simulink model "DF_DOB"  (R2020a)
settings: Solver=ode1  StartTime=0.0  StopTime=10  FixedStep=0.0001  RelTol=1e-3
undefined symbols (not defined in the file): A, B, C, D, SEA
libraries: simulink x5, cstblocks x4, cjt_library_models x1
settings Model: Creator=erimc  LastModifiedBy=Erim Can Ozcinar

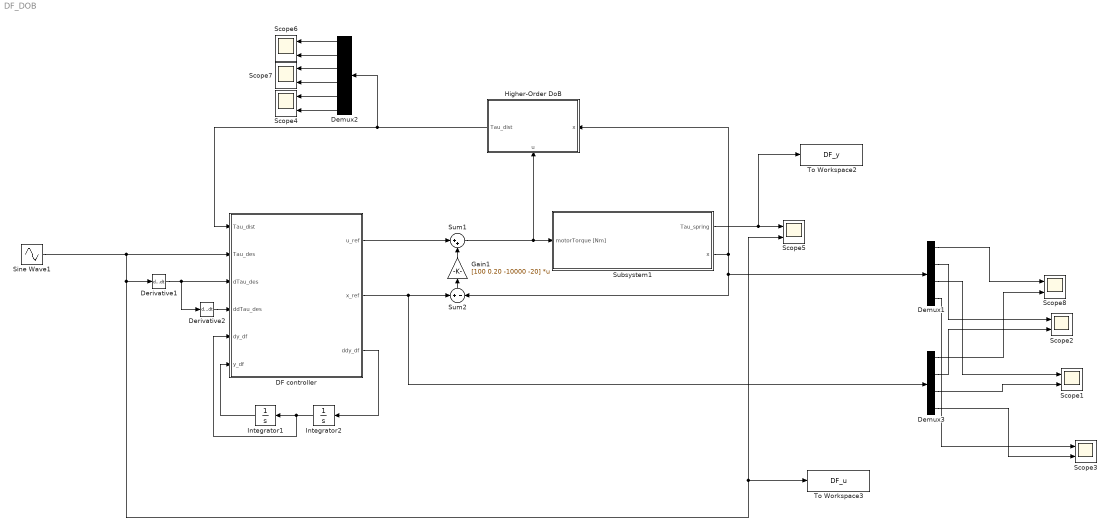
== system DF_DOB ==
  DF controller : MATLAB Function  TreatAsAtomicUnit=on
  Demux1 : Demux
  Demux2 : Demux  Outputs=6
  Demux3 : Demux
  Derivative1 : Derivative
  Derivative2 : Derivative
  Gain1 : Gain  Gain=[100 0.20 -10000 -20]  Multiplication=Matrix(K*u)
  Higher-Order DoB : Subsystem
      settings: PortSchema="{\"entries\":[{\"content\":{\"sides\":[{\"content\":{\"connectorIds\":[\"In1\"]},\"type\":\"ConnectorPlacement.EquallySpacedRectSide\",\"uuid\":\"033a9072-c968-43bf-9f71-6521bdc98383\"},{\"content\":{\"connectorIds\":[\"Out1\"],\"side\":\"RIGHT\"},\"type\":\"ConnectorPlacement.EquallySpacedRectSide\",\"uuid\":\"95ac0c33-e59d-4ac0-96cc-facae06806bd\"},{\"content\":{\"connectorIds\":[],\"side\":\"TOP\"},\"type\":\"ConnectorPlacement.EquallySpacedRectSide\",\"uuid\":\"4271cccc-922d-4503-b442-5df2d938e766\"},{\"content\":{\"connectorIds\":[\"In2\"],\"side\":\"BOTTOM\"},\"type\":\"ConnectorPlacement.EquallySpacedRectSide\",\"uuid\":\"8fe68d28-3df5-4424-a916-547538c04804\"}]},\"type\":\"ConnectorPlacement.EquallySpacedConnector\",\"uuid\":\"e60c16e9-b2aa-49f1-a4b3-0df40270c19e\"}],\"packageUris\":[\"http://schema.mathworks.com/mf0/Connector/19700101\"],\"version\":\"1.0\"}"
  Integrator1 : Integrator
  Integrator2 : Integrator
  Scope{1..8} (8 alike) : Scope  NumInputPorts=2
  Sine Wave1 : Sin  Amplitude=10  SampleTime=0
  Subsystem1 : Subsystem
  Sum1 : Sum  Inputs=|++
  Sum2 : Sum  Inputs=+|-
  To Workspace2 : ToWorkspace  VariableName=DF_y  SampleTime=-1
      settings: Save2DSignal=2-D array (concatenate along first dimension)
  To Workspace3 : ToWorkspace  VariableName=DF_u  SampleTime=-1
      settings: Save2DSignal=2-D array (concatenate along first dimension)
  wires:
  Integrator1/1 -> DF controller/6(y_df)
  Sum1/1 -> Subsystem1/1(motorTorque [Nm]), Higher-Order DoB/2(u)
  DF controller/2(x_ref) -> Sum2/1, Demux3/1
  DF controller/1(u_ref) -> Sum1/1
  Subsystem1/1(Tau_spring) -> To Workspace2/1, Scope5/1
  Demux1/1 -> Scope8/1
  Demux2/5 -> Scope4/1
  Subsystem1/2(x) -> Higher-Order DoB/1(x), Sum2/2, Demux1/1
  Demux3/3 -> Scope1/2
  Demux3/1 -> Scope8/2
  Demux3/2 -> Scope2/2
  Derivative1/1 -> DF controller/3(dTau_des), Derivative2/1
  Demux3/4 -> Scope3/2
  DF controller/3(ddy_df) -> Integrator2/1
  Demux1/2 -> Scope2/1
  Demux2/6 -> Scope4/2
  Demux2/2 -> Scope6/2
  Integrator2/1 -> DF controller/5(dy_df), Integrator1/1
  Demux1/3 -> Scope1/1
  Demux2/1 -> Scope6/1
  Demux1/4 -> Scope3/1
  Higher-Order DoB/1(Tau_dist) -> DF controller/1(Tau_dist), Demux2/1
  Demux2/3 -> Scope7/1
  Sine Wave1/1 -> DF controller/2(Tau_des), To Workspace3/1, Scope5/2, Derivative1/1
  Demux2/4 -> Scope7/2
  Gain1/1 -> Sum1/2
  Sum2/1 -> Gain1/1
  Derivative2/1 -> DF controller/4(ddTau_des)

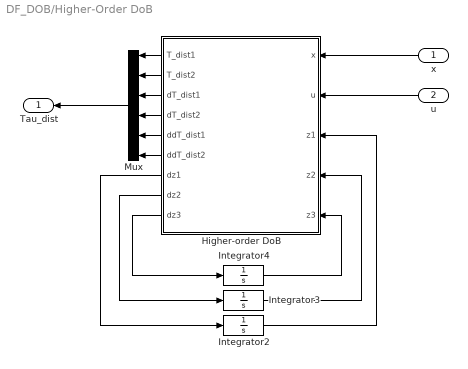
== system DF_DOB/Higher-Order DoB ==
  x : Inport
  u : Inport  Port=2
  Higher-order DoB : MATLAB Function  TreatAsAtomicUnit=on
  Integrator2 : Integrator
  Integrator3 : Integrator
  Integrator4 : Integrator
  Mux : Mux  Inputs=6
  Tau_dist : Outport
  wires:
  Integrator2/1 -> Higher-order DoB/3(z1)
  x/1 -> Higher-order DoB/1(x)
  u/1 -> Higher-order DoB/2(u)
  Integrator4/1 -> Higher-order DoB/5(z3)
  Integrator3/1 -> Higher-order DoB/4(z2)
  Higher-order DoB/1(T_dist1) -> Mux/1
  Higher-order DoB/2(T_dist2) -> Mux/2
  Higher-order DoB/3(dT_dist1) -> Mux/3
  Higher-order DoB/4(dT_dist2) -> Mux/4
  Higher-order DoB/5(ddT_dist1) -> Mux/5
  Higher-order DoB/6(ddT_dist2) -> Mux/6
  Mux/1 -> Tau_dist/1
  Higher-order DoB/8(dz2) -> Integrator3/1
  Higher-order DoB/7(dz1) -> Integrator2/1
  Higher-order DoB/9(dz3) -> Integrator4/1

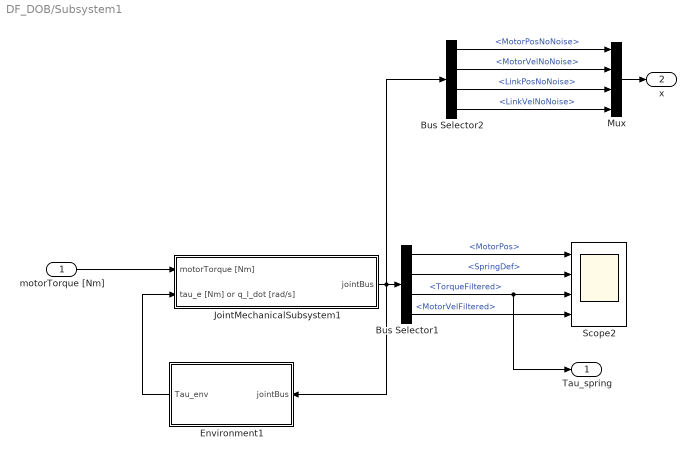
== system DF_DOB/Subsystem1 ==
  motorTorque [Nm] : Inport
  Bus Selector1 : BusSelector  OutputSignals=MotorPos,SpringDef,TorqueFiltered,MotorVelFiltered
  Bus Selector2 : BusSelector  OutputSignals=MotorPosNoNoise,MotorVelNoNoise,LinkPosNoNoise,LinkVelNoNoise
  Environment1 : Subsystem
  JointMechanicalSubsystem1 : Subsystem  AncestorBlock=cjt_library_models/Joint models/JointMechanicalSubsystem  mask(jointMechanicalSubsystem){jointObj=SEA, fc_vel=1000, fc_torque=1000, input_delay=0, output_delay=0, quantize=on, quantize_bits=19, input_noise_enabled=on, output_noise_enabled=on, var_u=0.021, var_y=1e-10}
      mask prompts: jointObj "Joint Object"; fc_vel "Velocity filter cut-off frequency [Hz]"; fc_torque "Torque filter cut-off frequency [Hz]"; input_delay "Motor torque input delay (num samples of Ts)"; output_delay "Output delay (num samples of Ts)"; quantize "Quantize measurements"; quantize_bits "Quantization bits"; input_noise_enabled "Enable input noise"; output_noise_enabled "Enable measurement noise"; var_u "Input noise variance"; var_y "Measurement noise variance"
      mask help:
      | This block implements the mechanical dynamics of the actuator.
      |
      | For more information, see the > Help <.
      mask init:
      | % Get linear dynamics matrices
      | [A, B, C, D, I, R, K] = jointObj.getDynamicsMatrices();
      | 
      | % Build B matrix for nonlinear components
      | B_nonlinear = [zeros([size(B,1)-size(I,1),1]); 1./diag(I)];
      | 
      | % Get other properties
      | Ts      = jointObj.Ts;
      | Ts_elec = jointObj.Ts_elec;
      | k_b     = jointObj.k_b;
      | k_t     = jointObj.k_t;
      | n       = jointObj.n;
      | d_gl    = jointObj.d_gl;
      | 
      | % Handle MATLAB function block
      | handleMatlabFunctionBlock(gcb, jointObj);
      | 
      | % If input delay is enabled, set the flag to 1
      | input_delay_enable = 0;
      | if (input_delay > 0)
      |     input_delay_enable = 1;
      | end
      | 
      | % If noise is disabled, overwrite the given variances
      | if (input_noise_enabled == 0)
      |     var_u = 0;
      | end
      | if (output_noise_enabled == 0)
      | 	var_y = 0;
      | end
      mask Help:
      | This block implements the mechanical dynamics of the actuator. Depending on the configuration in which the joint class was built, its dynamics are given by one of the variants provided by the toolbox (see model/linear/). If provided, the linear dynamics are enhanced with nonlinear components.
      | 
      | <b>Inputs</b>
      | <b>motorTorque</b>: Electromechanical motor torque provided on the rotor. An input delay can be added to this input (e.g. due to communication delays or a very simplified representation of electrical dynamics).
      | <b>tau_e or q_l_dot</b>: External interaction torque. Depending on the selected linear dynamics model of the joint, this is either the external torque acting on the load or the imposed load velocity (for fixed-output models).
      | 
      | <b>Outputs</b>
      | <b>jointBus</b>: The various variables and their measurements, with optional delays/noise/quantisation etc. For most outputs, several instances exist. Output variables ending in "NoNoise" denote physical quantities, without noise, filtering, or delays. All other variables are affected by noise and delays (if enabled). Lastly, variables ending in "Filtered" are also low-pass filtered, with cut-off frequency set in the mask.
      | 
      | <b>An important note with regards to output variables associated with torque.</b>
      | The "Torque" and "TorqueFiltered" are computed in the way torque is usually sensed by the control system; deflection times spring constant, i.e. only the stiffness contribution is considered, as usually the internal damping of the used flexible element (parameter d_gl) is very small. Hence, TorqueFiltered is used by the toolbox controllers as well.
      | However, as noted before, "TorqueNoNoise" denotes the physical quantity. This means that it includes the torque produced by internal damping of the elastic element (parameter d_gl).
      mask Callback quantize: toggleMaskFields(gcbh, 'quantize', 'quantize_bits');
      mask Callback input_noise_enabled: toggleMaskFields(gcbh, 'input_noise_enabled', 'var_u');
      mask Callback output_noise_enabled: toggleMaskFields(gcbh, 'output_noise_enabled', 'var_y');
  Mux : Mux
  Scope2 : Scope  NumInputPorts=4
  Tau_spring : Outport
  x : Outport  Port=2
  wires:
  Bus Selector1/2 -> Scope2/2  "<SpringDef>"
  Bus Selector1/3 -> Tau_spring/1, Scope2/3  "<TorqueFiltered>"
  JointMechanicalSubsystem1/1(jointBus) -> Bus Selector2/1, Environment1/1(jointBus), Bus Selector1/1
  Bus Selector1/1 -> Scope2/1  "<MotorPos>"
  motorTorque [Nm]/1 -> JointMechanicalSubsystem1/1(motorTorque [Nm])
  Bus Selector2/1 -> Mux/1  "<MotorPosNoNoise>"
  Bus Selector2/2 -> Mux/2  "<MotorVelNoNoise>"
  Bus Selector2/3 -> Mux/3  "<LinkPosNoNoise>"
  Bus Selector2/4 -> Mux/4  "<LinkVelNoNoise>"
  Mux/1 -> x/1
  Bus Selector1/4 -> Scope2/4  "<MotorVelFiltered>"
  Environment1/1(Tau_env) -> JointMechanicalSubsystem1/2(tau_e [Nm] or q_l_dot [rad/s])

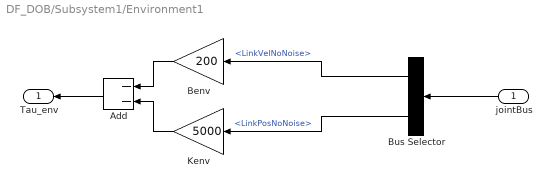
== system DF_DOB/Subsystem1/Environment1 ==
  jointBus : Inport
  Add : Sum  Inputs=--
  Benv : Gain  Gain=200
  Bus Selector : BusSelector  OutputSignals=LinkVelNoNoise,LinkPosNoNoise
  Kenv : Gain  Gain=5000
  Tau_env : Outport
  wires:
  Kenv/1 -> Add/2
  Benv/1 -> Add/1
  Add/1 -> Tau_env/1
  Bus Selector/1 -> Benv/1  "<LinkVelNoNoise>"
  Bus Selector/2 -> Kenv/1  "<LinkPosNoNoise>"
  jointBus/1 -> Bus Selector/1

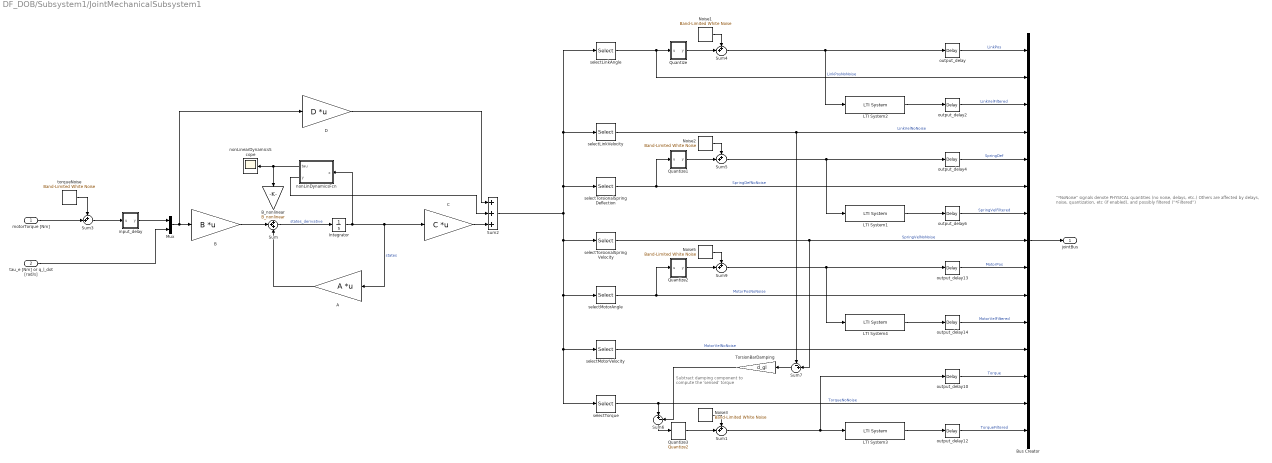
== system DF_DOB/Subsystem1/JointMechanicalSubsystem1 ==
  note: "*NoNoise" signals denote PHYSICAL quantities (no noise, delays, etc.)
      | Others are affected by delays, noise, quantization, etc (if enabled), and possibly filtered ("*Filtered")
  note: Subtract damping component to
      | compute the 'sensed' torque
  motorTorque [Nm] : Inport
  tau_e [Nm] or q_l_dot [rad/s] : Inport  Port=2
  A : Gain  Gain=A  Multiplication=Matrix(K*u)
  B : Gain  Gain=B  Multiplication=Matrix(K*u)
  B_nonlinear : Gain  Gain=B_nonlinear
  Bus Creator : BusCreator  Inputs=15
  C : Gain  Gain=C  Multiplication=Matrix(K*u)
  D : Gain  Gain=D  Multiplication=Matrix(K*u)
  Integrator : Integrator
  LTI System1 : cstblocks/LTI System  sys=c2d(tf([2*pi*fc_vel 0], [1 2*pi*fc_vel]), Ts, 'tustin')  IC=[]
  LTI System2 : cstblocks/LTI System  sys=c2d(tf([2*pi*fc_vel 0], [1 2*pi*fc_vel]), Ts, 'tustin')  IC=[]
  LTI System3 : cstblocks/LTI System  sys=c2d(tf([2*pi*fc_torque], [1 2*pi*fc_torque]), Ts, 'tustin')  IC=[]
  LTI System4 : cstblocks/LTI System  sys=c2d(tf([2*pi*fc_vel 0], [1 2*pi*fc_vel]), Ts, 'tustin')  IC=[]
  Mux : Mux  Inputs=2
  Noise1 : simulink/Sources/Band-Limited White Noise  Cov=var_y * Ts  Ts=Ts  seed=[3846513]
  Noise2 : simulink/Sources/Band-Limited White Noise  Cov=var_y * Ts  Ts=Ts  seed=[11563454]
  Noise3 : simulink/Sources/Band-Limited White Noise  Cov=sqrt(2) * var_y * Ts % sqrt(2) accounts for subtracting two encoders  Ts=Ts  seed=[960834]
  Noise5 : simulink/Sources/Band-Limited White Noise  Cov=var_y * Ts  Ts=Ts  seed=[24326]
  Quantize : Subsystem
  Quantize1 : Subsystem
  Quantize2 : Subsystem
  Quantize3 : cjt_library_models/Joint models/JointMechanicalSubsystem/Quantize2  SystemSampleTime=-1  Latency=0  AutoFrameSizeCalculation=off
  Sum : Sum  Inputs=+++
  Sum{1,3..5,9} (5 alike) : Sum  Inputs=++|
  Sum2 : Sum  Inputs=+++
  Sum6 : Sum  Inputs=|+-
  Sum7 : Sum  Inputs=-+|
  TorsionBarDamping : Gain  Gain=d_gl
  input_delay : Subsystem
  nonLinDynamicsFcn : MATLAB Function  TreatAsAtomicUnit=on
  nonLinearDynamicsScope : Scope
  output_delay{,2,4,6,10,12..14} (8 alike) : TransportDelay  DelayTime=output_delay * jointObj.Ts
  selectLinkAngle : Selector  NumberOfDimensions=2  InputPortWidth=3  IndexOptions=Index vector (dialog),Select all  Indices=3,1  OutputSizes=1,1
  selectLinkVelocity : Selector  NumberOfDimensions=2  InputPortWidth=3  IndexOptions=Index vector (dialog),Select all  Indices=6,1  OutputSizes=1,1
  selectMotorAngle : Selector  NumberOfDimensions=2  InputPortWidth=3  IndexOptions=Index vector (dialog),Select all  Indices=1,1  OutputSizes=1,1
  selectMotorVelocity : Selector  NumberOfDimensions=2  InputPortWidth=3  IndexOptions=Index vector (dialog),Select all  Indices=4,1  OutputSizes=1,1
  selectTorque : Selector  NumberOfDimensions=2  InputPortWidth=3  IndexOptions=Index vector (dialog),Select all  Indices=7,1  OutputSizes=1,1
  selectTorsionalSpringDeflection : Selector  NumberOfDimensions=2  InputPortWidth=3  IndexOptions=Index vector (dialog),Select all  Indices=2,1  OutputSizes=1,1
  selectTorsionalSpringVelocity : Selector  NumberOfDimensions=2  InputPortWidth=3  IndexOptions=Index vector (dialog),Select all  Indices=5,1  OutputSizes=1,1
  torqueNoise : simulink/Sources/Band-Limited White Noise  Cov=var_u * Ts  Ts=Ts  seed=[2435345645]
  jointBus : Outport
  wires:
  Sum6/1 -> Quantize3/1
  Noise3/1 -> Sum1/1
  Quantize3/1 -> Sum1/2
  Sum7/1 -> TorsionBarDamping/1
  TorsionBarDamping/1 -> Sum6/2
  C/1 -> Sum2/3
  D/1 -> Sum2/1
  Quantize2/1(y) -> Sum9/2
  Quantize1/1(y) -> Sum5/2
  Quantize/1(y) -> Sum4/2
  Sum1/1 -> LTI System3/1, output_delay10/1
  LTI System3/1 -> output_delay12/1
  tau_e [Nm] or q_l_dot [rad/s]/1 -> Mux/2
  Mux/1 -> B/1, D/1
  Sum9/1 -> output_delay13/1, LTI System4/1
  output_delay14/1 -> Bus Creator/11  "MotorVelFiltered"
  output_delay13/1 -> Bus Creator/9  "MotorPos"
  LTI System4/1 -> output_delay14/1
  Noise5/1 -> Sum9/1
  output_delay12/1 -> Bus Creator/15  "TorqueFiltered"
  selectTorque/1 -> Bus Creator/14, Sum6/1  "TorqueNoNoise"
  output_delay10/1 -> Bus Creator/13  "Torque"
  selectMotorVelocity/1 -> Bus Creator/12  "MotorVelNoNoise"
  selectMotorAngle/1 -> Bus Creator/10, Quantize2/1(u)  "MotorPosNoNoise"
  selectTorsionalSpringVelocity/1 -> Sum7/2, Bus Creator/8  "SpringVelNoNoise"
  output_delay6/1 -> Bus Creator/7  "SpringVelFiltered"
  selectTorsionalSpringDeflection/1 -> Bus Creator/6, Quantize1/1(u)  "SpringDefNoNoise"
  output_delay4/1 -> Bus Creator/5  "SpringDef"
  selectLinkVelocity/1 -> Sum7/1, Bus Creator/4  "LinkVelNoNoise"
  output_delay2/1 -> Bus Creator/3  "LinkVelFiltered"
  selectLinkAngle/1 -> Bus Creator/2, Quantize/1(u)  "LinkPosNoNoise"
  output_delay/1 -> Bus Creator/1  "LinkPos"
  A/1 -> Sum/3
  B/1 -> Sum/2
  Sum2/1 -> selectTorsionalSpringDeflection/1, selectLinkVelocity/1, selectLinkAngle/1, selectMotorAngle/1, selectMotorVelocity/1, selectTorque/1, selectTorsionalSpringVelocity/1
  Integrator/1 -> A/1, C/1, nonLinDynamicsFcn/1(x)  "states"
  motorTorque [Nm]/1 -> Sum3/2
  LTI System2/1 -> output_delay2/1
  Sum/1 -> Integrator/1  "states_derivative"
  LTI System1/1 -> output_delay6/1
  Noise1/1 -> Sum4/1
  Noise2/1 -> Sum5/1
  torqueNoise/1 -> Sum3/1
  Sum4/1 -> output_delay/1, LTI System2/1
  Sum5/1 -> output_delay4/1, LTI System1/1
  Sum3/1 -> input_delay/1(u)
  input_delay/1(y) -> Mux/1
  Bus Creator/1 -> jointBus/1
  nonLinDynamicsFcn/1(tau) -> B_nonlinear/1, nonLinearDynamicsScope/1
  nonLinDynamicsFcn/2(y) -> Sum2/2

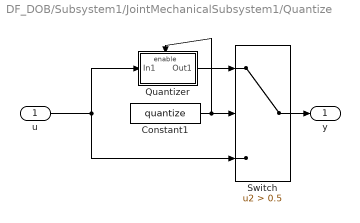
== system DF_DOB/Subsystem1/JointMechanicalSubsystem1/Quantize ==
  u : Inport
  Constant1 : Constant  Value=quantize
  Quantizer : Subsystem
  Switch : Switch  Criteria=u2 > Threshold  Threshold=0.5
  y : Outport
  wires:
  u/1 -> Quantizer/1(In1), Switch/3
  Constant1/1 -> Quantizer/Enable, Switch/2
  Switch/1 -> y/1
  Quantizer/1(Out1) -> Switch/1

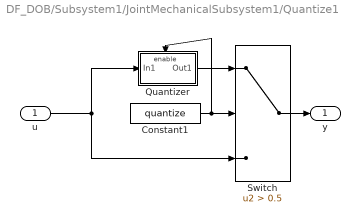
== system DF_DOB/Subsystem1/JointMechanicalSubsystem1/Quantize1 ==
  u : Inport
  Constant1 : Constant  Value=quantize
  Quantizer : Subsystem
  Switch : Switch  Criteria=u2 > Threshold  Threshold=0.5
  y : Outport
  wires:
  u/1 -> Quantizer/1(In1), Switch/3
  Constant1/1 -> Quantizer/Enable, Switch/2
  Switch/1 -> y/1
  Quantizer/1(Out1) -> Switch/1

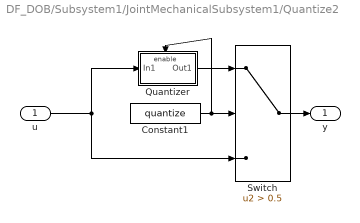
== system DF_DOB/Subsystem1/JointMechanicalSubsystem1/Quantize2 ==
  u : Inport
  Constant1 : Constant  Value=quantize
  Quantizer : Subsystem
  Switch : Switch  Criteria=u2 > Threshold  Threshold=0.5
  y : Outport
  wires:
  u/1 -> Quantizer/1(In1), Switch/3
  Constant1/1 -> Quantizer/Enable, Switch/2
  Switch/1 -> y/1
  Quantizer/1(Out1) -> Switch/1

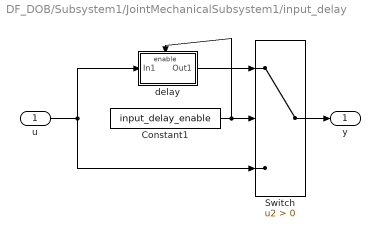
== system DF_DOB/Subsystem1/JointMechanicalSubsystem1/input_delay ==
  u : Inport
  Constant1 : Constant  Value=input_delay_enable
  Switch : Switch  Criteria=u2 > Threshold
  delay : Subsystem
  y : Outport
  wires:
  u/1 -> delay/1(In1), Switch/3
  Constant1/1 -> Switch/2, delay/Enable
  Switch/1 -> y/1
  delay/1(Out1) -> Switch/1

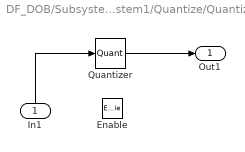
== system DF_DOB/Subsystem1/JointMechanicalSubsystem1/Quantize/Quantizer ==
  In1 : Inport
  Enable : EnablePort
  Quantizer : Quantizer  QuantizationInterval=1/(2^quantize_bits)
  Out1 : Outport
  wires:
  In1/1 -> Quantizer/1
  Quantizer/1 -> Out1/1

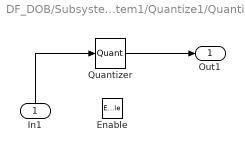
== system DF_DOB/Subsystem1/JointMechanicalSubsystem1/Quantize1/Quantizer ==
  In1 : Inport
  Enable : EnablePort
  Quantizer : Quantizer  QuantizationInterval=1/(2^quantize_bits)
  Out1 : Outport
  wires:
  In1/1 -> Quantizer/1
  Quantizer/1 -> Out1/1

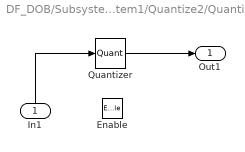
== system DF_DOB/Subsystem1/JointMechanicalSubsystem1/Quantize2/Quantizer ==
  In1 : Inport
  Enable : EnablePort
  Quantizer : Quantizer  QuantizationInterval=1/(2^quantize_bits)
  Out1 : Outport
  wires:
  In1/1 -> Quantizer/1
  Quantizer/1 -> Out1/1

== system DF_DOB/Subsystem1/JointMechanicalSubsystem1/input_delay/delay ==
  note: The delay value here is computed so that it is >0 when delay is DISABLED,
      | to avoid MATLAB throwing warnings unnecessarily.
  In1 : Inport
  Enable : EnablePort
  input_delay : TransportDelay  DelayTime=input_delay * jointObj.Ts + 1 - input_delay_enable  TransDelayFeedthrough=on
  Out1 : Outport
  wires:
  In1/1 -> input_delay/1
  input_delay/1 -> Out1/1

== matlab function DF_DOB/DF controller ==
  data: Tau_dist input; Tau_des input; u_ref output; dTau_des input; ddTau_des input; dy_df input; x_ref output; ddy_df output; y_df input
function [u_ref, x_ref, ddy_df] = fcn(Tau_dist, Tau_des, dTau_des, ddTau_des, dy_df, y_df)

Jm =  (2.781e-04); % kgm^2     *2
Bm = (1.5e-03);   % Nms/rad    *0.5
K = 5000;      %Nm/rad         *1.1
N = 100;        % -
Jl = 0.07;      % kgm^2        *1.5
Bl = 0.005;     % Nms/rad      *5

Kenv = 5000;
Benv = 200;

T_dist = Tau_dist(1:2);
dT_dist = Tau_dist(3:4);
ddT_dist = Tau_dist(5:6);

ddy_df = (N/Jl)*(Tau_des/K - T_dist(2)*N/K - (Bl + Benv)*dy_df/N - Kenv*y_df/(N*N));
dddy_df = (N/Jl)*(dTau_des/K - dT_dist(2)*N/K - (Bl + Benv)*ddy_df/N - Kenv*dy_df/(N*N));
ddddy_df = (N/Jl)*(ddTau_des/K - ddT_dist(2)*N/K - (Bl + Benv)*dddy_df/N - Kenv*ddy_df/(N*N));

x1 = (Jl*ddy_df) + (Bl + Benv)*dy_df + (K + Kenv)*y_df/N + (N*N*T_dist(2)/K); % qm
x2 = (Jl*dddy_df) + (Bl + Benv)*ddy_df + (K + Kenv)*dy_df/N + (N*N*dT_dist(2)/K); % dqm
x3 = K*y_df/(N*N); % ql
x4 = K*dy_df/(N*N); % dql

x_ref = [x1; x2; x3; x4]; % Referance states

p1 = Jm*Jl;
p2 = Jm*(Bl + Benv) + Jl*Bm;
p3 = K*Jl/(N*N) + (K + Kenv)*Jm/N + Bm*(Bl + Benv);
p4 = K*(Bl + Benv)/(N*N) + (K + Kenv)*Bm/N;
p5 = K*Kenv/(N*N);
d_total = N*N*Jm*ddT_dist(2)/K + N*N*Bm*dT_dist(2)/K + T_dist(2) + T_dist(1);

u_ref = p1*ddddy_df + p2*dddy_df + p3*ddy_df + p4*dy_df + d_total; % + p5*y_df

== matlab function DF_DOB/Higher-Order DoB/Higher-order DoB ==
  data: x input; u input; T_dist1 output; T_dist2 output; dT_dist1 output; dT_dist2 output; ddT_dist1 output; ddT_dist2 output; z1 input; z2 input; z3 input; dz1 output; dz2 output; dz3 output
function [T_dist1, T_dist2, dT_dist1, dT_dist2, ddT_dist1, ddT_dist2, dz1, dz2, dz3] = fcn(x, u, z1, z2, z3)

Jm =  (2.781e-04); % kgm^2     *2
Bm = (1.5e-03);   % Nms/rad    *0.5
K = 5000;      %Nm/rad         *1.1
N = 100;        % -
Jl = 0.07;      % kgm^2        *1.5
Bl = 0.005;     % Nms/rad      *5
Kenv = 5000;
Benv = 200;

%% For states x = [qm dqm ql dql]
A = [    0            1         0          0;...
    -K/(Jm*N*N)    -Bm/Jm    K/(Jm*N)      0;...
         0            0         0          1;...
     K/(Jl*N)         0    -(K+Kenv)/Jl  -(Bl+Benv)/Jl];
 
B = [0; 1/Jm; 0; 0];

%% Higher-order DOB

f = 300*2*pi; % DoB frequency
L1 = 3*f;
L2 = 3*f^2;
L3 = f^3;

dz1 = -L1*z1 + z2 + L1*(A*x + B*u + L1*x) - L2*x;
dz2 = -L2*z1 + z3 + L2*(A*x + B*u + L1*x) - L3*x;
dz3 = -L3*z1 + L3*(A*x + B*u + L1*x);

T_dist = z1 - L1*x;
dT_dist = z2 - L2*x;
ddT_dist = z3 - L3*x;

T_dist1 = T_dist(2)*Jm; 
T_dist2 = T_dist(4)*Jl;
dT_dist1 = dT_dist(2)*Jm; 
dT_dist2 = dT_dist(4)*Jl;
ddT_dist1 = ddT_dist(2)*Jm; 
ddT_dist2 = ddT_dist(4)*Jl;

% Tau_dist = [T_dist(2); T_dist(4); dT_dist(2); dT_dist(4); ddT_dist(2); ddT_dist(4)];

== matlab function DF_DOB/Subsystem1/JointMechanicalSubsystem1/nonLinDynamicsFcn ==
  data: tau output; x input; y output
function [tau, y] = nonLinDynamics(x)
%#codegen

params.a_CU = 0.003900;
params.c_CU = 380.000000;
params.c_FE = 460.000000;
params.diam = 98.000000;
params.len = 166.000000;
params.m = 3.400000;
params.I_m = 0.000278;
params.I_g = 0.000000;
params.I_l = 0.070000;
params.k_g = 0.000000;
params.k_b = 5000.000000;
params.d_m = 0.001500;
params.d_g = 0.000000;
params.d_l = 0.005000;
params.d_m_n = 0.001500;
params.d_g_n = 0.000000;
params.d_l_n = 0.005000;
params.d_mg = 0.000000;
params.d_gl = 0.000000;
params.d_cm = 0.073950;
params.d_cg = 0.000000;
params.d_cl = 0.000000;
params.d_cm_n = 0.069810;
params.d_cg_n = 0.000000;
params.d_cl_n = 0.000000;
params.d_s = 0.000000;
params.v_s = 0.000000;
params.rip_types = [];
params.rip_a1 = [];
params.rip_a2 = [];
params.rip_f = [];
params.n = 100.000000;
params.k_t = 0.102000;
params.r = 0.370000;
params.x = 0.000400;
params.p = 12.000000;
params.v_0 = 48.000000;
params.i_p = 36.000000;
params.dq_p = 411.548600;
params.r_th1 = 1.637200;
params.r_th2 = 15.292500;
params.T_thw = 90.014100;
params.T_thm = 3781.168300;
params.Tmp_WMax = 155.000000;
params.Tmp_ANom = 25.000000;
params.name = 'sea_Pomegranate';
params.paramName = 'sea_param';
params.modelName = 'sea';
%params.nonlinearModelName = {'coulomb', 'viscous_asym'}; % Cell arrays are not supported for code generation.
params.electricalModelName = 'electric_dyn_2';
params.Ts = 0.001000;
params.Ts_elec = 0.000100;

[tau_1, y_1] = coulomb(params,x);
[tau_2, y_2] = viscous_asym(params,x);
tau = tau_1 +tau_2;
y = y_1 +y_2;
	end
